simulink model "Butter"  (R2021a)
settings: Solver=VariableStepAuto  StartTime=0.0  StopTime=10.0  RelTol=1e-3
undefined symbols (not defined in the file or in its folder): ap2, bp2
settings Model: Creator=simao  LastModifiedBy=simao

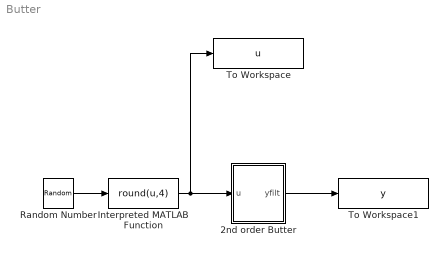
== system Butter ==
  2nd order Butter : Subsystem
  Interpreted MATLAB Function : MATLABFcn  MATLABFcn=round(u,4)
  Random Number : RandomNumber  SampleTime=0.02
  To Workspace : ToWorkspace  VariableName=u  SaveFormat=Timeseries  SampleTime=0.02
  To Workspace1 : ToWorkspace  VariableName=y  SaveFormat=Timeseries  SampleTime=0.02
  wires:
  Random Number/1 -> Interpreted MATLAB Function/1
  Interpreted MATLAB Function/1 -> 2nd order Butter/1(u), To Workspace/1
  2nd order Butter/1(yfilt) -> To Workspace1/1

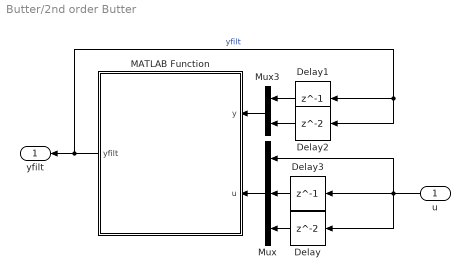
== system Butter/2nd order Butter ==
  u : Inport
  Delay : Delay
  Delay1 : Delay  DelayLength=1  SampleTime=0.02
  Delay2 : Delay
  Delay3 : Delay  DelayLength=1  SampleTime=0.02
  MATLAB Function : MATLAB Function  TreatAsAtomicUnit=on
  Mux : Mux  Inputs=3
  Mux3 : Mux  Inputs=2
  yfilt : Outport
  wires:
  Mux3/1 -> MATLAB Function/1(y)
  Mux/1 -> MATLAB Function/2(u)
  MATLAB Function/1(yfilt) -> Delay1/1, Delay2/1, yfilt/1  "yfilt"
  Delay/1 -> Mux/3
  Delay3/1 -> Mux/2
  u/1 -> Mux/1, Delay3/1, Delay/1
  Delay1/1 -> Mux3/1
  Delay2/1 -> Mux3/2

== matlab function Butter/2nd order Butter/MATLAB Function ==
  data: y input; u input; yfilt output; bp2 parameter; ap2 parameter
function yfilt = filtit(y,u, bp2, ap2)
b = bp2;
a = ap2;
yfilt = 0;
for i=1:length(u)
   yfilt = yfilt + b(i)*u(i);
end

for i=2:length(y)+1
   yfilt = yfilt - a(i)*y(i-1); 
end

yfilt = yfilt/a(1);

end
